simulink model "fig2_49_simulink"  (R2021b)
settings: Solver=ode45  StartTime=0.0  StopTime=100  RelTol=1e-3  EnableMultiTasking=on
undefined symbols (not defined in the file or in its folder): c
settings Model: Creator=One Informatic  LastModifiedBy=One Informatic
settings DataIOCC: LimitDataPoints=on  SaveFormat=Array  SignalLoggingSaveFormat=ModelDataLogs  ReturnWorkspaceOutputs=off  SignalLoggingName=sigsOut
settings DebuggingCC: SaveWithParameterizedLinksMsg=none  UnderspecifiedInitializationDetection=Classic  MergeDetectMultiDrivingBlocksExec=none  SignalResolutionControl=TryResolveAllWithWarning  MultiTaskDSMMsg=warning  MultiTaskCondExecSysMsg=none
settings HardwareCC: ProdBitPerPointer=32  ProdBitPerSizeT=32  ProdBitPerPtrDiffT=32  ProdLargestAtomicFloat=None  ProdIntDivRoundTo=Undefined  ProdEndianess=Unspecified  ProdWordSize=32  ProdHWDeviceType=32-bit Generic  TargetUnknown=on
settings ModelReferenceCC: PropagateSignalLabelsOutOfModel=off
settings GRTTargetCC: CombineOutputUpdateFcns=off  GRTInterface=on
settings ConfigComp: CovMetricSettings=dw  CovSaveCumulativeToWorkspaceVar=on  CovSaveSingleToWorkspaceVar=on

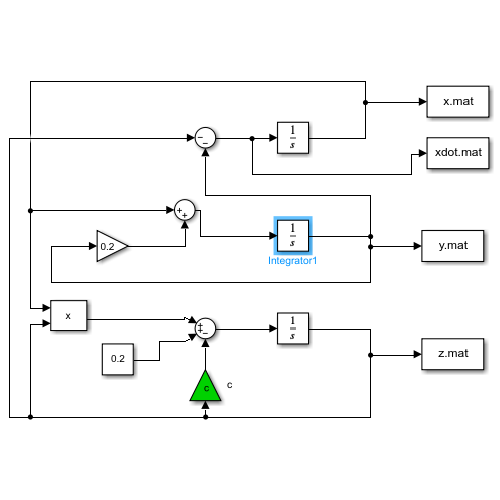
[thumbnail: Simulink's stored preview of the top-level diagram]
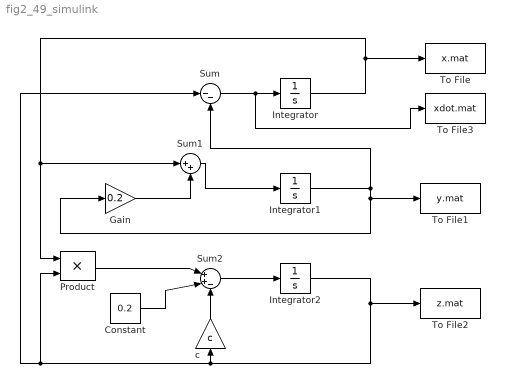
== system fig2_49_simulink ==
  Constant : Constant  Value=0.2
  Gain : Gain  Gain=0.2  SaturateOnIntegerOverflow=on  OutDataTypeStr=Inherit: Same as input  ParamDataTypeStr=Inherit: Same as input
  Integrator : Integrator  InitialCondition=0.3
  Integrator1 : Integrator  InitialCondition=0.23
  Integrator2 : Integrator  InitialCondition=0.8
  Product : Product  SaturateOnIntegerOverflow=on  OutDataTypeStr=Inherit: Same as first input
  Sum : Sum  Inputs=|--  SaturateOnIntegerOverflow=on
  Sum1 : Sum  Inputs=|++  SaturateOnIntegerOverflow=on
  Sum2 : Sum  Inputs=|++-  SaturateOnIntegerOverflow=on
  To File : ToFile  Filename=x.mat  MatrixName=x  SampleTime=0.01
  To File1 : ToFile  Filename=y.mat  MatrixName=y  SampleTime=0.01
  To File2 : ToFile  Filename=z.mat  MatrixName=z  SampleTime=0.01
  To File3 : ToFile  Filename=xdot.mat  MatrixName=xdot  SampleTime=0.01
  c : Gain  Gain=c  SaturateOnIntegerOverflow=on  OutDataTypeStr=Inherit: Same as input  ParamDataTypeStr=Inherit: Same as input
  wires:
  Sum/1 -> Integrator/1, To File3/1
  Sum1/1 -> Integrator1/1
  Sum2/1 -> Integrator2/1
  Constant/1 -> Sum2/2
  c/1 -> Sum2/3
  Integrator2/1 -> c/1, Product/2, Sum/1, To File2/1
  Product/1 -> Sum2/1
  Integrator1/1 -> Gain/1, To File1/1, Sum/2
  Gain/1 -> Sum1/2
  Integrator/1 -> To File/1, Product/1, Sum1/1
